simulink model "mass_spring_damper_transfer_function"  (R2022a)
settings: Solver=ode45  StartTime=0.0  StopTime=Sim_Time  MaxStep=0.01  RelTol=1e-3  EnableMultiTasking=on
undefined symbols (not defined in the file): b, F, k, M
settings Model: Creator=dzr3qn  LastModifiedBy=Dr. Ryan Aly
settings SolverCC: AlgebraicLoopSolver=TrustRegion
settings DataIOCC: LimitDataPoints=on  SaveFormat=Array  ReturnWorkspaceOutputs=off
settings OptimizationCC: LifeSpan=inf
settings DebuggingCC: SolverPrmCheckMsg=warning  UnconnectedInputMsg=warning  UnconnectedOutputMsg=warning  UnconnectedLineMsg=warning  SFUnexpectedBacktrackingDiag=warning  SFNoUnconditionalDefaultTransitionDiag=warning  SFExecutionAtInitializationDiag=none  SFMachineParentedDataDiag=warning  ArithmeticOperatorsInVariantConditions=warning
settings HardwareCC: ProdBitPerPointer=32  ProdBitPerSizeT=32  ProdBitPerPtrDiffT=32  ProdLargestAtomicFloat=None  ProdIntDivRoundTo=Undefined  ProdEndianess=Unspecified  ProdWordSize=32  ProdHWDeviceType=32-bit Generic
settings ModelReferenceCC: PropagateSignalLabelsOutOfModel=off
settings SFSimCC: SimUseLocalCustomCode=off  CustomCodeUndefinedFunction=UseInterfaceOnly
settings RTWCC: RTWUseLocalCustomCode=off
settings CodeAppCC: StateflowObjectComments=on
settings GRTTargetCC: TargetLangStandard=C89/C90 (ANSI)
settings ConfigComp: CovMetricSettings=dw  CovSaveCumulativeToWorkspaceVar=on  CovSaveSingleToWorkspaceVar=on  CovExternalEMLEnable=off  CovSFcnEnable=off

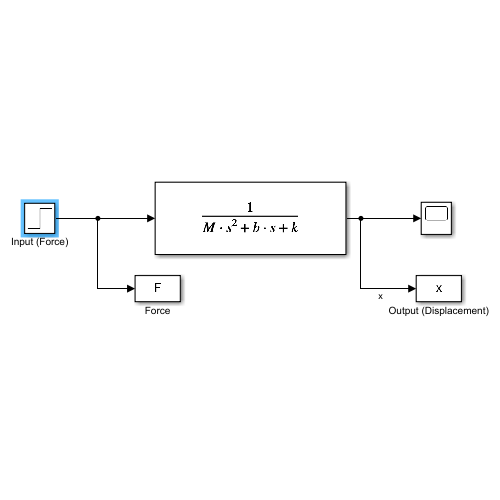
[thumbnail: Simulink's stored preview of the top-level diagram]
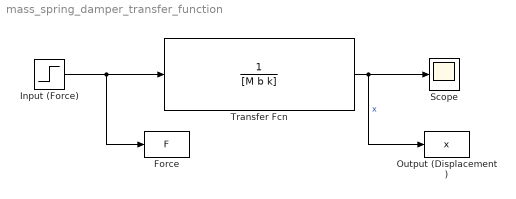
== system mass_spring_damper_transfer_function ==
  Force : ToWorkspace  VariableName=F  SaveFormat=Timeseries  SampleTime=-1
  Input (Force) : Step  After=F  SampleTime=0  ZeroCross=off
  Output (Displacement) : ToWorkspace  VariableName=x  SaveFormat=Timeseries  SampleTime=-1
  Scope : Scope
  Transfer Fcn : TransferFcn  Denominator=[M b k]
  wires:
  Input (Force)/1 -> Force/1, Transfer Fcn/1
  Transfer Fcn/1 -> Output (Displacement)/1, Scope/1  "x"
